simulink model "kinEq_sim"  (R2020a)
settings: Solver=FixedStepDiscrete  StartTime=0.0  StopTime=11  FixedStep=TS  RelTol=1e-3  EnableMultiTasking=on
PostLoadFcn:
  | params
model workspace (MAT data in the model file):
  Ia = 0.1
  Id = 0.25
  Pa = 5
  Pd = 9
  TS = 0.01
undefined symbols (not defined in the file): DiscIntNeverNeededParam, L, r, sigbuilder_block, StartTheta, StartX, StartY
libraries: simulink_extras x3
settings Model: EnablePacing=on  Creator=mgovinda  LastModifiedBy=mmarathe
settings DataIOCC: LimitDataPoints=on  SaveFormat=Array  ReturnWorkspaceOutputs=off
settings OptimizationCC: LifeSpan=inf
settings DebuggingCC: SFUnexpectedBacktrackingDiag=warning  SFNoUnconditionalDefaultTransitionDiag=warning  SFExecutionAtInitializationDiag=none  ArithmeticOperatorsInVariantConditions=warning
settings HardwareCC: ProdBitPerPointer=32  ProdBitPerSizeT=32  ProdBitPerPtrDiffT=32  ProdLargestAtomicFloat=None  ProdIntDivRoundTo=Undefined  ProdEndianess=Unspecified  ProdWordSize=32  ProdHWDeviceType=32-bit Generic
settings ModelReferenceCC: PropagateSignalLabelsOutOfModel=off
settings SFSimCC: SimUseLocalCustomCode=off  CustomCodeUndefinedFunction=UseInterfaceOnly
settings RTWCC: RTWUseLocalCustomCode=off
settings CodeAppCC: StateflowObjectComments=on
settings GRTTargetCC: TargetLangStandard=C89/C90 (ANSI)
settings ConfigComp: CovMetricSettings=dw  CovSaveCumulativeToWorkspaceVar=on  CovSaveSingleToWorkspaceVar=on  CovExternalEMLEnable=off

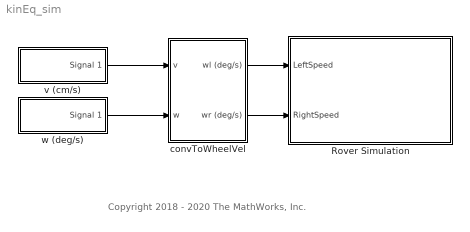
== system kinEq_sim ==
  note: Copyright 2018 - 2020 The MathWorks, Inc.
  Rover Simulation : Subsystem
  convToWheelVel : Subsystem
  v (cm/s) : Subsystem  Tag=STV Subsys  LoadFcn=sigbuilder_block('load',[2.25 144.75 600.75 275.25 ]);  StartFcn=sigbuilder_block('start');  StopFcn=sigbuilder_block('stop');  ClipboardFcn=sigbuilder_block('clipboard');  mask(Sigbuilder block){tuvar=[0:10]}
      mask help: Simulink:masks:SigbuilderBlock_MD
      mask init:
      | if ~strcmp(get_param(bdroot(gcbh),'SimulationStatus'),'stopped') tuvar = sigbuilder_block('maskInit'); end
      settings: CopyFcn=sigbuilder_block('copy');  DeleteFcn=sigbuilder_block('delete');  ModelCloseFcn=sigbuilder_block('modelClose');  PreSaveFcn=sigbuilder_block('preSave');  PauseFcn=sigbuilder_block('pause');  ContinueFcn=sigbuilder_block('continue');  NameChangeFcn=sigbuilder_block('namechange');  OpenFcn=sigbuilder_block('open',[347.25 153 600.75 275.25 ]);  CloseFcn=sigbuilder_block('close');
      mask Display: plot(0, 0, 100, 100,[2, 2, 32, 32, 2], [68, 8, 8, 68, 68],[32, 2], [38, 38], [32, 19, 2],[53, 60, 44], [32, 17, 17, 2],[16, 16, 31, 31]);txt = getActiveGroup(gcbh);text(2, 100, txt,'verticalAlignment', 'top');
  w (deg/s) : Subsystem  Tag=STV Subsys  LoadFcn=sigbuilder_block('load',[210.75 142.5 475.5 277.5 ]);  StartFcn=sigbuilder_block('start');  StopFcn=sigbuilder_block('stop');  ClipboardFcn=sigbuilder_block('clipboard');  mask(Sigbuilder block){tuvar=[0:10]}
      mask help: Simulink:masks:SigbuilderBlock_MD
      mask init:
      | if ~strcmp(get_param(bdroot(gcbh),'SimulationStatus'),'stopped') tuvar = sigbuilder_block('maskInit'); end
      settings: CopyFcn=sigbuilder_block('copy');  DeleteFcn=sigbuilder_block('delete');  ModelCloseFcn=sigbuilder_block('modelClose');  PreSaveFcn=sigbuilder_block('preSave');  PauseFcn=sigbuilder_block('pause');  ContinueFcn=sigbuilder_block('continue');  NameChangeFcn=sigbuilder_block('namechange');  OpenFcn=sigbuilder_block('open',[170.25 180.75 475.5 277.5 ]);  CloseFcn=sigbuilder_block('close');
      mask Display: plot(0, 0, 100, 100,[2, 2, 32, 32, 2], [68, 8, 8, 68, 68],[32, 2], [38, 38], [32, 19, 2],[53, 60, 44], [32, 17, 17, 2],[16, 16, 31, 31]);txt = getActiveGroup(gcbh);text(2, 100, txt,'verticalAlignment', 'top');
  wires:
  convToWheelVel/1(wl (deg/s)) -> Rover Simulation/1(LeftSpeed)
  convToWheelVel/2(wr (deg/s)) -> Rover Simulation/2(RightSpeed)
  v (cm/s)/1(Signal 1) -> convToWheelVel/1(v)
  w (deg/s)/1(Signal 1) -> convToWheelVel/2(w)

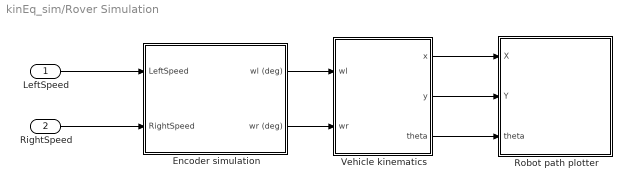
== system kinEq_sim/Rover Simulation ==
  LeftSpeed : Inport
  RightSpeed : Inport  Port=2
  " Encoder simulation" : Subsystem
  Robot path plotter : Subsystem
  Vehicle kinematics : Subsystem
  wires:
  Vehicle kinematics/1(x) -> Robot path plotter/1(X)
  Vehicle kinematics/2(y) -> Robot path plotter/2(Y)
  Vehicle kinematics/3(theta) -> Robot path plotter/3(theta)
  LeftSpeed/1 -> " Encoder simulation"/1(LeftSpeed)
  RightSpeed/1 -> " Encoder simulation"/2(RightSpeed)
  " Encoder simulation"/1(wl (deg)) -> Vehicle kinematics/1(wl)
  " Encoder simulation"/2(wr (deg)) -> Vehicle kinematics/2(wr)

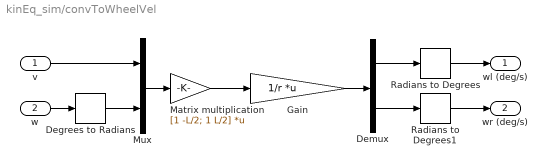
== system kinEq_sim/convToWheelVel ==
  v : Inport
  w : Inport  Port=2
  " Gain" : Gain  Gain=1/r  Multiplication=Matrix(K*u)
  Degrees to Radians : simulink_extras/Transformations/Degrees to Radians
  Demux : Demux  Outputs=2
  Matrix multiplication : Gain  Gain=[1 -L/2; 1 L/2]  Multiplication=Matrix(K*u)
  Mux : Mux  Inputs=2
  Radians to Degrees : simulink_extras/Transformations/Radians to Degrees
  Radians to Degrees1 : simulink_extras/Transformations/Radians to Degrees
  wl (deg/s) : Outport  VectorParamsAs1DForOutWhenUnconnected=off
  wr (deg/s) : Outport  Port=2  VectorParamsAs1DForOutWhenUnconnected=off
  wires:
  " Gain"/1 -> Demux/1
  Matrix multiplication/1 -> " Gain"/1
  v/1 -> Mux/1
  Mux/1 -> Matrix multiplication/1
  Demux/1 -> Radians to Degrees/1
  Demux/2 -> Radians to Degrees1/1
  w/1 -> Degrees to Radians/1
  Radians to Degrees/1 -> wl (deg/s)/1
  Radians to Degrees1/1 -> wr (deg/s)/1
  Degrees to Radians/1 -> Mux/2

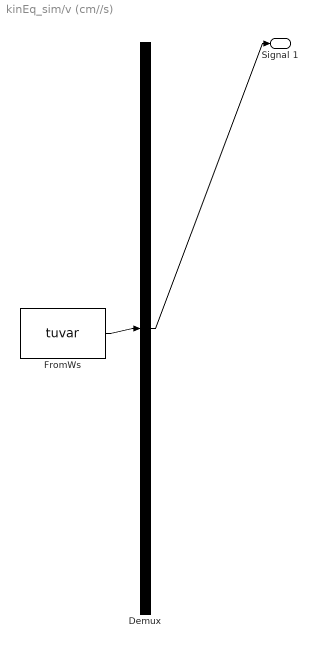
== system kinEq_sim/v (cm//s) ==
  Demux : Demux  Tag=STV Demux  Outputs=1
      settings: DisplayOption=none
  FromWs : FromWorkspace  Tag=STV FromWs  VariableName=tuvar
      SigBuilderData=|
      | common.afterFinalStr = 'Extrapolate'
      | common.sampleTime = 0
      | dataSet.timeRange = [0 10]
      | dataSet.name = 'Group 1'
      | sbobj.Groups.Name = 'Group 1'
      | sbobj.Groups.Signals.Name = 'Signal 1'
      | sbobj.Groups.Signals.XData = [0 5 5 6 10]
      | sbobj.Groups.Signals.YData = [10 10 0 0 0]
  Signal 1 : Outport  Tag=STV Outport  VectorParamsAs1DForOutWhenUnconnected=off
  wires:
  Demux/1 -> Signal 1/1
  FromWs/1 -> Demux/1

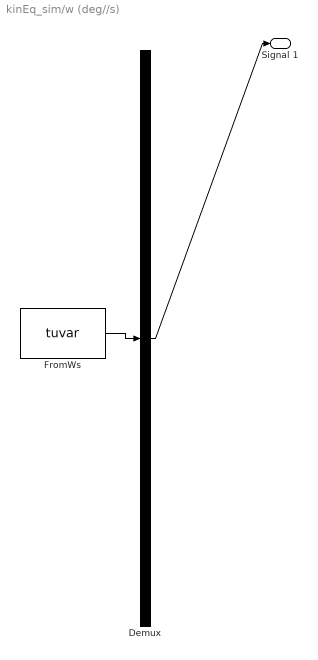
== system kinEq_sim/w (deg//s) ==
  Demux : Demux  Tag=STV Demux  Outputs=1
      settings: DisplayOption=none
  FromWs : FromWorkspace  Tag=STV FromWs  VariableName=tuvar
      SigBuilderData=|
      | common.afterFinalStr = 'Extrapolate'
      | common.sampleTime = 0
      | dataSet.timeRange = [0 11]
      | dataSet.name = 'Group 1'
      | sbobj.Groups.Name = 'Group 1'
      | sbobj.Groups.Signals.Name = 'Signal 1'
      | sbobj.Groups.Signals.XData = [0 5 5 10 10 11]
      | sbobj.Groups.Signals.YData = [0 0 72 72 0 0]
      | sbobj.Groups.TimeRange = [0 11]
  Signal 1 : Outport  Tag=STV Outport  VectorParamsAs1DForOutWhenUnconnected=off
  wires:
  FromWs/1 -> Demux/1
  Demux/1 -> Signal 1/1

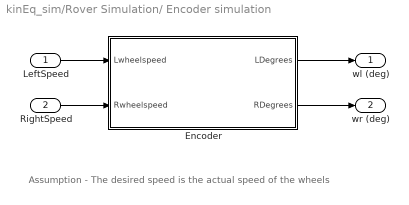
== system kinEq_sim/Rover Simulation/ Encoder simulation ==
  note: Assumption - The desired speed is the actual speed of the wheels
  LeftSpeed : Inport
  RightSpeed : Inport  Port=2
  Encoder : Subsystem
  wl (deg) : Outport  VectorParamsAs1DForOutWhenUnconnected=off
  wr (deg) : Outport  Port=2  VectorParamsAs1DForOutWhenUnconnected=off
  wires:
  Encoder/1(LDegrees) -> wl (deg)/1
  Encoder/2(RDegrees) -> wr (deg)/1
  RightSpeed/1 -> Encoder/2(Rwheelspeed)
  LeftSpeed/1 -> Encoder/1(Lwheelspeed)

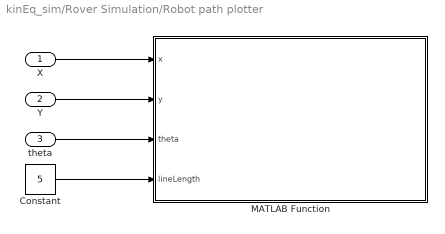
== system kinEq_sim/Rover Simulation/Robot path plotter ==
  X : Inport
  Y : Inport  Port=2
  theta : Inport  Port=3
  Constant : Constant  Value=5
  "MATLAB Function " : MATLAB Function  TreatAsAtomicUnit=on
  wires:
  Constant/1 -> "MATLAB Function "/4(lineLength)
  X/1 -> "MATLAB Function "/1(x)
  Y/1 -> "MATLAB Function "/2(y)
  theta/1 -> "MATLAB Function "/3(theta)

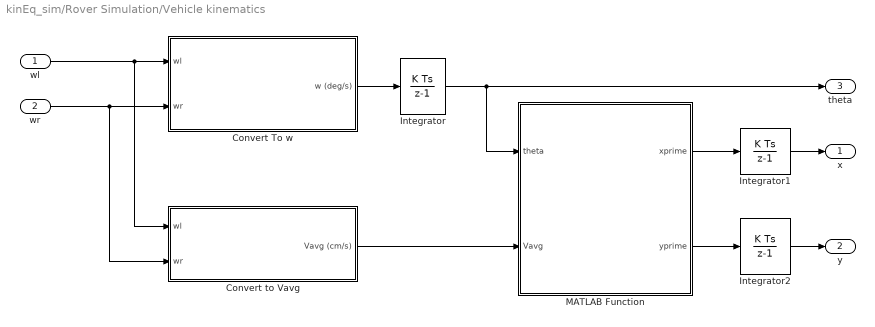
== system kinEq_sim/Rover Simulation/Vehicle kinematics ==
  wl : Inport
  wr : Inport  Port=2
  Convert To w : Subsystem
  Convert to Vavg : Subsystem
  Integrator : DiscreteIntegrator  gainval=1  InitialCondition=StartTheta  SampleTime=-1  ICPrevOutput=DiscIntNeverNeededParam  ICPrevScaledInput=DiscIntNeverNeededParam
  Integrator1 : DiscreteIntegrator  gainval=1  InitialCondition=StartX  SampleTime=-1  ICPrevOutput=DiscIntNeverNeededParam  ICPrevScaledInput=DiscIntNeverNeededParam
  Integrator2 : DiscreteIntegrator  gainval=1  InitialCondition=StartY  SampleTime=-1  ICPrevOutput=DiscIntNeverNeededParam  ICPrevScaledInput=DiscIntNeverNeededParam
  "MATLAB Function " : MATLAB Function  TreatAsAtomicUnit=on
  x : Outport  VectorParamsAs1DForOutWhenUnconnected=off
  y : Outport  Port=2  VectorParamsAs1DForOutWhenUnconnected=off
  theta : Outport  Port=3  VectorParamsAs1DForOutWhenUnconnected=off
  wires:
  "MATLAB Function "/1(xprime) -> Integrator1/1
  "MATLAB Function "/2(yprime) -> Integrator2/1
  Integrator1/1 -> x/1
  Integrator2/1 -> y/1
  Integrator/1 -> theta/1, "MATLAB Function "/1(theta)
  wl/1 -> Convert to Vavg/1(wl), Convert To w/1(wl)
  wr/1 -> Convert to Vavg/2(wr), Convert To w/2(wr)
  Convert to Vavg/1(Vavg (cm/s)) -> "MATLAB Function "/2(Vavg)
  Convert To w/1(w (deg/s)) -> Integrator/1

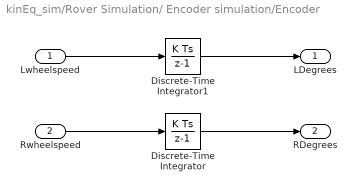
== system kinEq_sim/Rover Simulation/ Encoder simulation/Encoder ==
  Lwheelspeed : Inport
  Rwheelspeed : Inport  Port=2
  Discrete-Time Integrator : DiscreteIntegrator  SampleTime=-1  ICPrevOutput=DiscIntNeverNeededParam  ICPrevScaledInput=DiscIntNeverNeededParam
  Discrete-Time Integrator1 : DiscreteIntegrator  SampleTime=-1  ICPrevOutput=DiscIntNeverNeededParam  ICPrevScaledInput=DiscIntNeverNeededParam
  LDegrees : Outport  VectorParamsAs1DForOutWhenUnconnected=off
  RDegrees : Outport  Port=2  VectorParamsAs1DForOutWhenUnconnected=off
  wires:
  Rwheelspeed/1 -> Discrete-Time Integrator/1
  Lwheelspeed/1 -> Discrete-Time Integrator1/1
  Discrete-Time Integrator/1 -> RDegrees/1
  Discrete-Time Integrator1/1 -> LDegrees/1

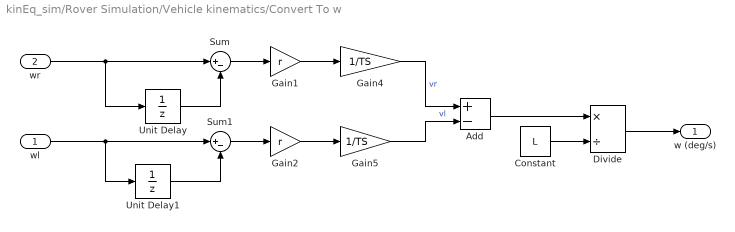
== system kinEq_sim/Rover Simulation/Vehicle kinematics/Convert To w ==
  wl : Inport
  wr : Inport  Port=2
  Add : Sum  Inputs=+-
  Constant : Constant  Value=L
  Divide : Product  Inputs=*/
  Gain1 : Gain  Gain=r
  Gain2 : Gain  Gain=r
  Gain4 : Gain  Gain=1/TS
  Gain5 : Gain  Gain=1/TS
  Sum : Sum  Inputs=|+-
  Sum1 : Sum  Inputs=|+-
  Unit Delay : UnitDelay  SampleTime=-1  HasFrameUpgradeWarning=on
  Unit Delay1 : UnitDelay  SampleTime=-1  HasFrameUpgradeWarning=on
  w (deg/s) : Outport  VectorParamsAs1DForOutWhenUnconnected=off
  wires:
  Unit Delay1/1 -> Sum1/2
  Sum1/1 -> Gain2/1
  wl/1 -> Sum1/1, Unit Delay1/1
  wr/1 -> Sum/1, Unit Delay/1
  Sum/1 -> Gain1/1
  Unit Delay/1 -> Sum/2
  Gain1/1 -> Gain4/1
  Gain2/1 -> Gain5/1
  Add/1 -> Divide/1
  Constant/1 -> Divide/2
  Gain4/1 -> Add/1  "vr"
  Gain5/1 -> Add/2  "vl"
  Divide/1 -> w (deg/s)/1

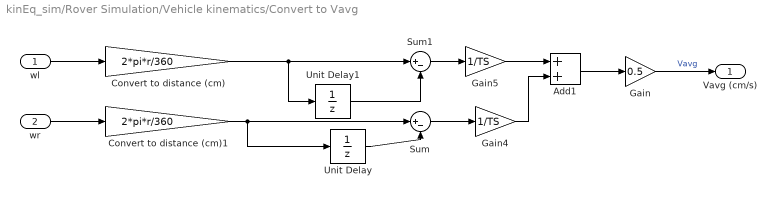
== system kinEq_sim/Rover Simulation/Vehicle kinematics/Convert to Vavg ==
  wl : Inport
  wr : Inport  Port=2
  Add1 : Sum
  Convert to distance (cm) : Gain  Gain=2*pi*r/360
  Convert to distance (cm)1 : Gain  Gain=2*pi*r/360
  Gain : Gain  Gain=0.5
  Gain4 : Gain  Gain=1/TS
  Gain5 : Gain  Gain=1/TS
  Sum : Sum  Inputs=|+-
  Sum1 : Sum  Inputs=|+-
  Unit Delay : UnitDelay  SampleTime=-1  HasFrameUpgradeWarning=on
  Unit Delay1 : UnitDelay  SampleTime=-1  HasFrameUpgradeWarning=on
  Vavg (cm/s) : Outport  VectorParamsAs1DForOutWhenUnconnected=off
  wires:
  Gain/1 -> Vavg (cm/s)/1  "Vavg"
  Add1/1 -> Gain/1
  Unit Delay/1 -> Sum/2
  Sum/1 -> Gain4/1
  wr/1 -> Convert to distance (cm)1/1
  Gain4/1 -> Add1/2
  Gain5/1 -> Add1/1
  Sum1/1 -> Gain5/1
  Unit Delay1/1 -> Sum1/2
  wl/1 -> Convert to distance (cm)/1
  Convert to distance (cm)/1 -> Unit Delay1/1, Sum1/1
  Convert to distance (cm)1/1 -> Unit Delay/1, Sum/1

== matlab function kinEq_sim/Rover Simulation/Robot path plotter/MATLAB Function  ==
  data: x input; y input; theta input; lineLength input; StartX parameter; StartY parameter; StartTheta parameter
function plotRobot(x,y,theta,lineLength, StartX, StartY, StartTheta)

% Create persistent variables for the figure windows
persistent h h1 h2;

if isempty(h)
    % Set up the initial figure window to display the initial position of
    % the rover
    h = figure('name','Map of the Robot');
    h1 = plot(StartX,StartY,'bo');
    hold on
    xlim([0 100])
    ylim([0 100])
    
    % Update the plot to show the heading of the rover
    xp = [StartX StartX+lineLength*cosd(StartTheta)];
    yp = [StartY StartY+lineLength*sind(StartTheta)];
    h2 = plot(xp,yp,'b');
    hold off
end

% Visualize the rover's path and heading
set(h1,'xdata',x,'ydata',y)
xp = [x x+lineLength*cosd(theta)];
yp = [y y+lineLength*sind(theta)];
set(h2,'xdata',xp,'ydata',yp)
drawnow('limitrate')

== matlab function kinEq_sim/Rover Simulation/Vehicle kinematics/MATLAB Function  ==
  settings: updateMethod=DISCRETE  sampleTime=TS
  data: xprime output; yprime output; theta input; Vavg input
function [xprime, yprime] = vehiclesPath(theta, Vavg)
%#codegen

% Implement the equation for the real-world location of the rover
xprime = Vavg*cosd(theta);
yprime = Vavg*sind(theta);
